simulink model "forney_test"  (R2020b)
settings: Solver=FixedStepAuto  StartTime=0.0  StopTime=10  FixedStep=1  RelTol=1e-3
settings Model: SILPILModeSetting=veronly  ExtModeTrigDuration=2  Creator=tcbir  LastModifiedBy=tcbir
settings OptimizationCC: EnhancedBackFolding=on  PassReuseOutputArgsAs=Individual arguments  ZeroExternalMemoryAtStartup=off  ZeroInternalMemoryAtStartup=off  MaxStackSize=64  OptimizeBlockOrder=speed  DifferentSizesBufferReuse=on  OptimizationCustomize=off  EfficientTunableParamExpr=on
settings DebuggingCC: ParameterTunabilityLossMsg=error
settings HardwareCC: ProdBitPerInt=16  ProdBitPerPointer=16  ProdBitPerSizeT=16  ProdBitPerPtrDiffT=16  ProdLargestAtomicFloat=None  ProdWordSize=8  ProdHWDeviceType=Atmel->AVR  UseEmbeddedCoderFeatures=off  UseSimulinkCoderFeatures=off
settings RTWCC: Description=Embedded Coder  SystemTargetFile=ert.tlc  HardwareBoard=Arduino Mega 2560  TemplateMakefile=ert_default_tmf  Toolchain=Arduino AVR
settings CodeAppCC: ForceParamTrailComments=on  IgnoreCustomStorageClasses=off  OperatorAnnotations=on  SimulinkDataObjDesc=on  SFDataObjDesc=on  InsertBlockDesc=on
settings ERTTargetCC: SupportContinuousTime=on  SupportNonInlinedSFcns=on  SupportVariableSizeSignals=on  ExtModeStaticAllocSize=2048

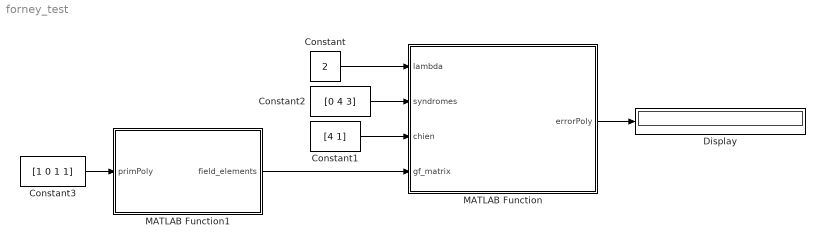
== system forney_test ==
  Constant : Constant  Value=2
  Constant1 : Constant  Value=[4 1]
  Constant2 : Constant  Value=[0 4 3]
  Constant3 : Constant  Value=[1 0 1 1]
  Display : Display
  MATLAB Function : MATLAB Function  TreatAsAtomicUnit=on
  MATLAB Function1 : MATLAB Function  TreatAsAtomicUnit=on
  wires:
  MATLAB Function1/1(field_elements) -> MATLAB Function/4(gf_matrix)
  Constant3/1 -> MATLAB Function1/1(primPoly)
  Constant/1 -> MATLAB Function/1(lambda)
  Constant2/1 -> MATLAB Function/2(syndromes)
  Constant1/1 -> MATLAB Function/3(chien)
  MATLAB Function/1(errorPoly) -> Display/1

== matlab function forney_test/MATLAB Function1 ==
  data: primPoly input; field_elements output
% GenerateGF2m: generates the selected Galois Field element. The inputs should be the
% order m and the coefficients of an appropriate primitive polynomial. The generated field,
% in either binary or power notation, may be a calling parameter for each of the other
% functions. Hint: I strongly suggest that you input the coefficients in “power” notation,
% with the highest order power on the left

function field_elements  = GenerateGF2m(primPoly) %primPoly in power notation, highest order on left

m = 3;
% hard coded size of retrun matrices and gf mtrix because simulink
% whines about variable output size. Havent figured out how to fix it
% ask laberge
gf = zeros(8, 3); %there are 2^m field elements
field_elements = zeros(8, 3); %there are 2^m field elements

gfIndx = 2; %gfIndx(1) holds initial state 
numShifts = (2^m) - 1;
s_reg = zeros(1,int8(m));
s_reg(end) = 1; %rightmost element of init shr is 1
gf(1, :) = 0;%write the contents of the init shift register to the matrix of gf elements
gf(2, :) = s_reg;
for i = 2:numShifts %number of shifts corresponds to power of primitive element
    carryOut = s_reg(1);%save the value to be wrapped
    for i0 = 1:numel(s_reg)-1
        if primPoly(i0 + 1) == 1
            s_reg(i0) = xor(carryOut, s_reg(i0 + 1));
        else
            s_reg(i0) = s_reg(i0 + 1);
        end
    end
    s_reg(end) = carryOut;
    gf(i+1,:) = s_reg; %add the newly shifted register to the gf matrix
end
field_elements = gf;
end

== matlab function forney_test/MATLAB Function ==
  data: lambda input; errorPoly output; syndromes input; chien input; gf_matrix input
function errorPoly  = ForneyAlgorithmRS(lambda,syndromes,chien,gf_matrix)
%function to establish and find the roots of the Error Evaluator Polynomial
%omega = lambda*(s + 1)modx^
%multiply lambda by the syndrome + 1
%msg = 'Executing Forney Algorithm...';
%disp(msg);

indx = 1;
while lambda(indx) == -1
    indx = indx + 1;
end

lambda = lambda(indx:numel(lambda));

modNum = 2^numel(gf_matrix(1,:)) - 1;

%flip syndromes (because it is reversed in berlekamp)
s_flipped = -1*ones(1,(numel(syndromes) + 1));
s_flipped(1:numel(syndromes)) = flip(syndromes);
s_flipped(end) = 0;
p = PolyMultGF2m(lambda, s_flipped, gf_matrix);

%ignore all terms with degree than r = n - k = 2t
[n, k] = size(gf_matrix);
[row_p, col_p] = size(p);
r = (n - 1) - k;
ix = col_p - r + 2;
omega = p(ix:end); %modulus
deriv = -1*ones(1,numel(omega));

%printo = ['Omega: [', num2str(omega(:).'), ']'];
%disp(printo);

%compute formal derivative
errorPolyTemp = -1*ones(1,chien(1)+1); 
errorPoly = -1*ones(1,chien(1)+1); 

xpwr = 1;
derivIndx = numel(deriv);
for j = (numel(lambda) - 1):-1:1
    if xpwr == 1
        deriv(derivIndx) = lambda(j);
    elseif mod(xpwr, 2) == 0 %if it's even, the GF addition cancels
        deriv(derivIndx) = -1;
    else
        deriv(derivIndx) = lambda(j); %shift right
    end
    derivIndx = derivIndx - 1;
    xpwr = xpwr + 1;
end

% errorPoly = -1*ones(1,chien(1)+1); 

%sub each Chien value into Forney's expression
for i0 = 1:numel(chien) %start at highest power
   intPoly = -1*ones(1,numel(omega));    
   errorIndx = numel(errorPoly) - (chien(i0));
   negative = modNum - chien(i0); 
   coef = chien(i0) - deriv(end); %subtract outside alpha from denominator alpha
   
   xpwr = numel(omega) - 1;
   for i1 = 1:numel(omega) %for each term in omega
        intPoly(i1) = xpwr * negative; %evaluate x at the exponent
        intPoly(i1) = intPoly(i1) + omega(i1); %add that to the coefficient power (multiply)
        xpwr = xpwr - 1;
   end
   
   %distribute the new outside alpha and do mod
   for i2 = 1:numel(intPoly)
       intPoly(i2) = intPoly(i2) + coef;
       intPoly(i2) = mod(intPoly(i2), modNum);
   end
   
   %combine terms and solve
   for i3 = 1:numel(intPoly) %for each term
        for i4 = i3 + 1:numel(intPoly) %check the other terms to cancel
            if numel(intPoly) > 1
                if intPoly(i4) == intPoly(i3)
                    intPoly(i4) = [];
                    intPoly(i3) = [];
                end
             end
       end
   end
   
   if numel(intPoly) ~= 1
       eval1 = intPoly(1);
       for i5 = 2:numel(intPoly)
           eval1 = AddGF2m(eval1, intPoly(i5), gf_matrix);
       end
   else
       eval1 = intPoly(1);
   end
   
   errorPolyTemp(errorIndx) = eval1;
   errorPoly = errorPolyTemp(1, :);
%    eval = EvalPolyGF2m(omega, negative, gf_matrix); %eval omega at negative chien value
%    product = MultGF2m(chien(i0), eval, gf_matrix); %multiply result by positive chien value
%    derivEval = EvalPolyGF2m(deriv, negative, gf_matrix); %divide that by deriv evaluated at negative chien 
%    errorPoly(errorIndx) = PolyDivGF2m(product, derivEval, gf_matrix);
end
%print = ['Error pattern: [', num2str(errorPoly(:).'), ']'];
%disp(print);
end
